simulink subsystem "trajectory_tracking_non_linear_sub"  (R2022b)
settings: Solver=VariableStepAuto  StartTime=0.0  StopTime=10.0  RelTol=1e-3
libraries: dspsigops x1
settings Model: Creator=Edp  LastModifiedBy=Edp

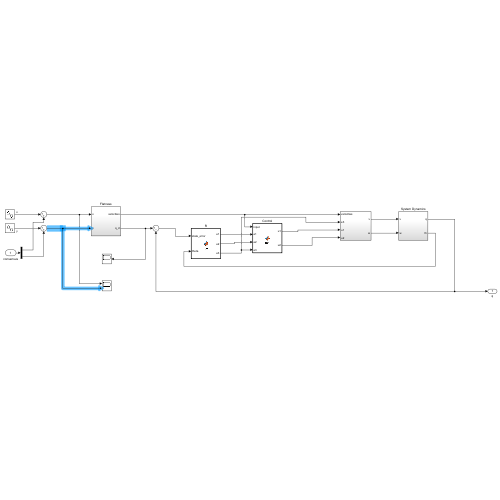
[thumbnail: Simulink's stored preview of the top-level diagram]
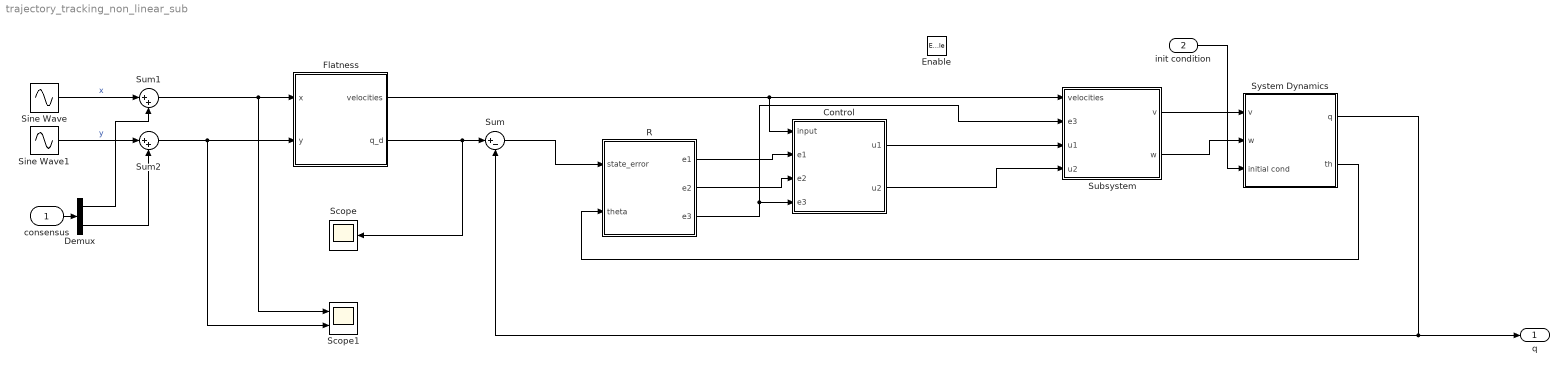
== system trajectory_tracking_non_linear_sub ==
  consensus : Inport
  init condition : Inport  Port=2
  Enable : EnablePort
  Control : MATLAB Function  TreatAsAtomicUnit=on
  Demux : Demux  Outputs=2
  Flatness : Subsystem
  R : MATLAB Function  TreatAsAtomicUnit=on
  Scope : Scope
  Scope1 : Scope  NumInputPorts=2
  Sine Wave : Sin  SampleTime=0
  Sine Wave1 : Sin  Phase=pi/2  SampleTime=0
  Subsystem : Subsystem
  Sum : Sum  Inputs=|+-
  Sum1 : Sum  Inputs=|++
  Sum2 : Sum  Inputs=|++
  System Dynamics : Subsystem
  q : Outport
  wires:
  Subsystem/2(w) -> System Dynamics/2(w)
  Subsystem/1(v) -> System Dynamics/1(v)
  Flatness/1(velocities) -> Control/1(input), Subsystem/1(velocities)
  Sine Wave/1 -> Sum1/1  "x"
  Control/1(u1) -> Subsystem/3(u1)
  R/3(e3) -> Subsystem/2(e3), Control/4(e3)
  Flatness/2(q_d) -> Scope/1, Sum/1
  Sum/1 -> R/1(state_error)
  R/1(e1) -> Control/2(e1)
  Control/2(u2) -> Subsystem/4(u2)
  R/2(e2) -> Control/3(e2)
  consensus/1 -> Demux/1
  Demux/1 -> Sum1/2
  Sum1/1 -> Scope1/1, Flatness/1(x)
  Sine Wave1/1 -> Sum2/1  "y"
  Demux/2 -> Sum2/2
  Sum2/1 -> Scope1/2, Flatness/2(y)
  init condition/1 -> System Dynamics/3(initial cond)
  System Dynamics/2(th) -> R/2(theta)
  System Dynamics/1(q) -> q/1, Sum/2

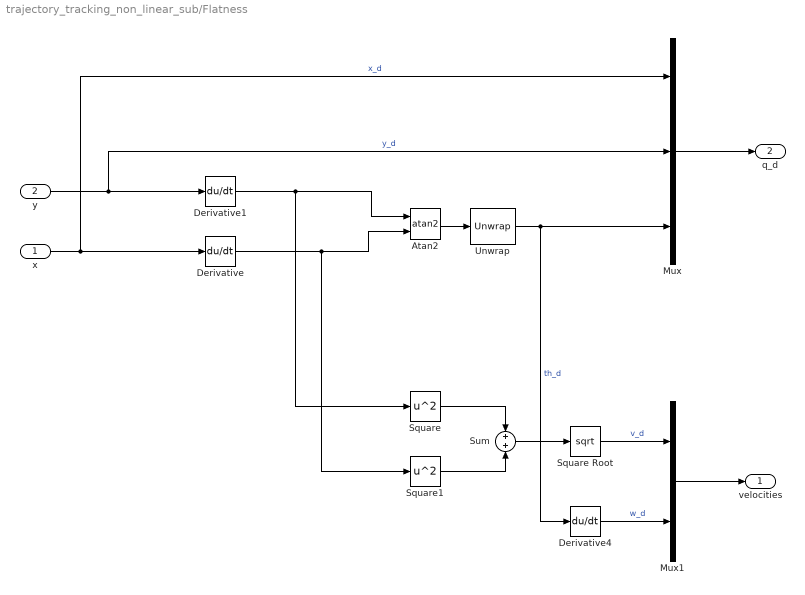
== system trajectory_tracking_non_linear_sub/Flatness ==
  x : Inport
  y : Inport  Port=2
  Atan2 : Trigonometry  Operator=atan2
  Derivative : Derivative
  Derivative1 : Derivative
  Derivative4 : Derivative
  Mux : Mux  Inputs=3
  Mux1 : Mux  Inputs=2
  Square : Math  Operator=square
  Square Root : Sqrt
  Square1 : Math  Operator=square
  Sum : Sum  Inputs=+|+
  Unwrap : dspsigops/Unwrap  tol=pi  running=off
  velocities : Outport
  q_d : Outport  Port=2
  wires:
  Derivative/1 -> Square1/1, Atan2/2
  x/1 -> Derivative/1, Mux/1  "x_d"
  Derivative1/1 -> Square/1, Atan2/1
  Atan2/1 -> Unwrap/1
  y/1 -> Derivative1/1, Mux/2  "y_d"
  Mux/1 -> q_d/1
  Square/1 -> Sum/1
  Square1/1 -> Sum/2
  Sum/1 -> Square Root/1
  Mux1/1 -> velocities/1
  Square Root/1 -> Mux1/1  "v_d"
  Derivative4/1 -> Mux1/2  "w_d"
  Unwrap/1 -> Derivative4/1, Mux/3  "th_d"

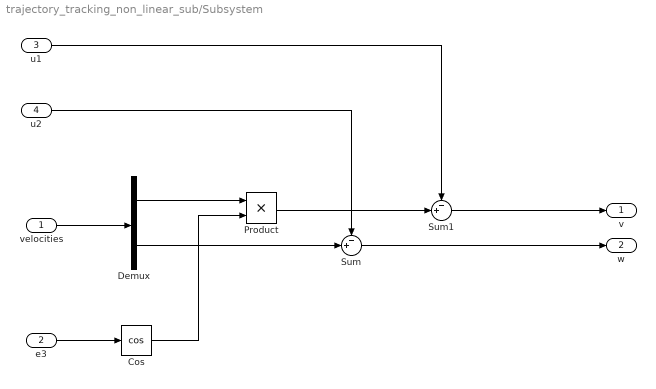
== system trajectory_tracking_non_linear_sub/Subsystem ==
  velocities : Inport
  e3 : Inport  Port=2
  u1 : Inport  Port=3
  u2 : Inport  Port=4
  Cos : Trigonometry  Operator=cos
  Demux : Demux  Outputs=2
  Product : Product
  Sum : Sum  Inputs=-+|
  Sum1 : Sum  Inputs=-+|
  v : Outport
  w : Outport  Port=2
  wires:
  velocities/1 -> Demux/1
  e3/1 -> Cos/1
  Demux/1 -> Product/1
  Cos/1 -> Product/2
  Demux/2 -> Sum/2
  u2/1 -> Sum/1
  Product/1 -> Sum1/2
  u1/1 -> Sum1/1
  Sum1/1 -> v/1
  Sum/1 -> w/1

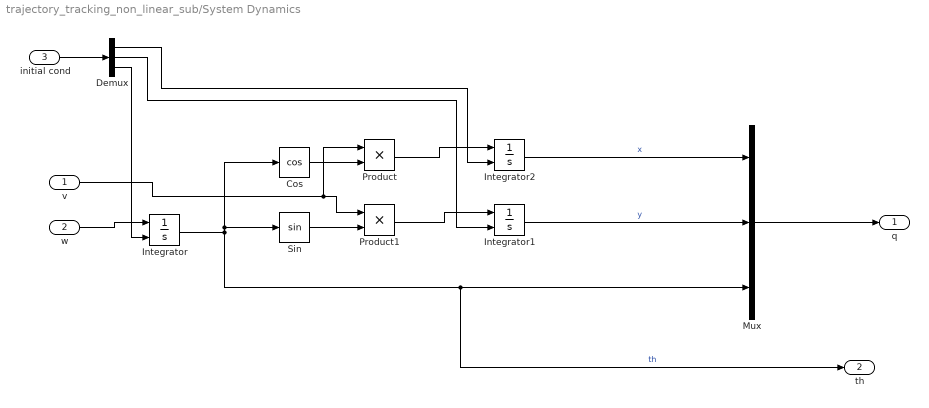
== system trajectory_tracking_non_linear_sub/System Dynamics ==
  v : Inport
  w : Inport  Port=2
  initial cond : Inport  Port=3
  Cos : Trigonometry  Operator=cos
  Demux : Demux  Outputs=3
  Integrator : Integrator  InitialConditionSource=external
  Integrator1 : Integrator  InitialConditionSource=external
  Integrator2 : Integrator  InitialConditionSource=external
  Mux : Mux  Inputs=3
  Product : Product
  Product1 : Product
  Sin : Trigonometry
  q : Outport
  th : Outport  Port=2
  wires:
  Demux/3 -> Integrator/2
  Demux/2 -> Integrator1/2
  Demux/1 -> Integrator2/2
  initial cond/1 -> Demux/1
  Cos/1 -> Product/2
  Integrator2/1 -> Mux/1  "x"
  Sin/1 -> Product1/2
  Integrator1/1 -> Mux/2  "y"
  Integrator/1 -> Mux/3, th/1, Sin/1, Cos/1  "th"
  Product1/1 -> Integrator1/1
  Product/1 -> Integrator2/1
  v/1 -> Product1/1, Product/1
  w/1 -> Integrator/1
  Mux/1 -> q/1

== matlab function trajectory_tracking_non_linear_sub/Control ==
  data: input input; e1 input; u1 output; e2 input; e3 input; u2 output
function [u1, u2]= fcn(input, e1, e2, e3)

csi = 1/sqrt(2);
a = 10;
b = 2;
v_d  = input(1);
w_d = input(2);


if abs(input(1)) < 1e-4
    if input(1) >= 0 
        input(1) = 1e-4;
    else 
        input(1) = -1e-4;
    end
end


k1 = 2*csi*sqrt(b*v_d + w_d^2);
k2 = b;
k3 = k1;

K = [-k1, 0, 0; 0 -k2*v_d*sin(e3)/e3, -k3];
e = [e1; e2; e3];

u = K*e;

u1 = u(1);
u2 = u(2);

== matlab function trajectory_tracking_non_linear_sub/R ==
  data: state_error input; e1 output; theta input; e2 output; e3 output
function [e1, e2, e3]= fcn(state_error, theta)

R = [cos(theta), sin(theta), 0; -sin(theta), cos(theta), 0; 0, 0, 1];

e = R*state_error;

e1 = e(1);
e2 = e(2);
e3 = e(3);
